simulink model "mrsMultiRobotAvoidance"  (R2018a)
settings: Solver=FixedStepAuto  StartTime=0.0  StopTime=inf  FixedStep=sampleTime  RelTol=1e-3
PreLoadFcn:
  | % Simulation parameters
  | load exampleMap
  | sampleTime = 0.05;
  | 
  | % Robot parameters
  | wheelRadius = 0.025;
  | robotRadius = 0.35;
  | 
  | % Lidar parameters
  | sensorOffset = [0,0];
  | scanAngles = linspace(-pi/2,pi/2,9)';
  | maxRange = 5;
libraries: mobileRoboticsLib x10
settings Model: EnablePacing=on  Creator=scastro  LastModifiedBy=scastro

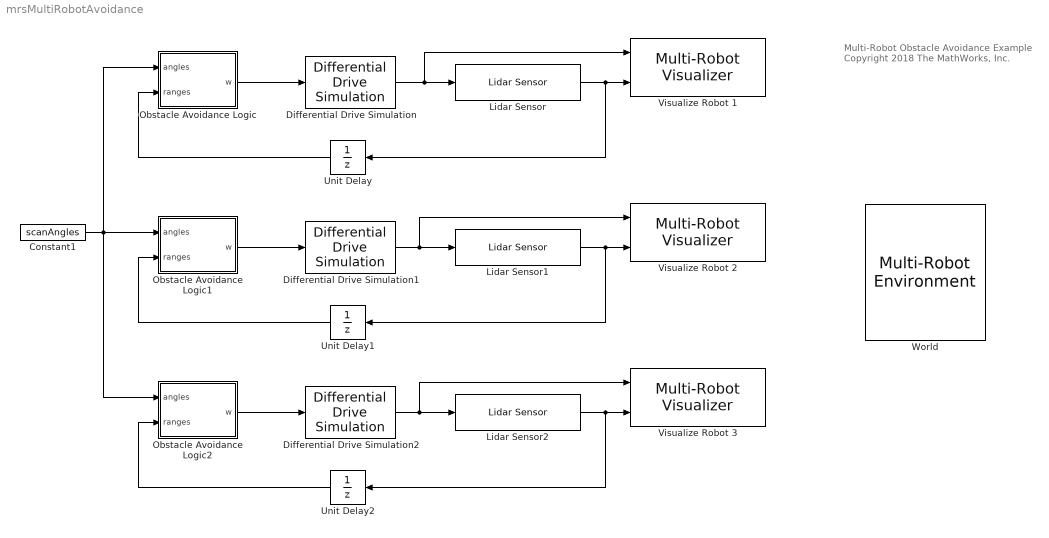
== system mrsMultiRobotAvoidance ==
  note: Multi-Robot Obstacle
      | Avoidance Example
      |
      | Copyright 2018 The MathWorks, Inc.
  Constant1 : Constant  Value=scanAngles
  Differential Drive Simulation : mobileRoboticsLib/Kinematic Models/Differential Drive/Differential Drive Simulation  OverrideUsingVariant=mode==2  wheelRadius=wheelRadius  wheelBase=robotRadius  initX=4  initY=4  initAngle=0  Ts=sampleTime
      settings: SourceProductName=Mobile Robotics Simulation Toolbox
  Differential Drive Simulation1 : mobileRoboticsLib/Kinematic Models/Differential Drive/Differential Drive Simulation  OverrideUsingVariant=mode==2  wheelRadius=wheelRadius  wheelBase=robotRadius  initX=8  initY=8  initAngle=pi/2  Ts=sampleTime
      settings: SourceProductName=Mobile Robotics Simulation Toolbox
  Differential Drive Simulation2 : mobileRoboticsLib/Kinematic Models/Differential Drive/Differential Drive Simulation  OverrideUsingVariant=mode==2  wheelRadius=wheelRadius  wheelBase=robotRadius  initX=7.5  initY=3  initAngle=-pi/4  Ts=sampleTime
      settings: SourceProductName=Mobile Robotics Simulation Toolbox
  Lidar Sensor : mobileRoboticsLib/Environments/Lidar Sensor  mapName=map  sensorOffset=sensorOffset  scanAngles=scanAngles  maxRange=maxRange  isMultiRobot=on  robotIdx=1
      settings: SourceProductName=Mobile Robotics Simulation Toolbox
  Lidar Sensor1 : mobileRoboticsLib/Environments/Lidar Sensor  mapName=map  sensorOffset=sensorOffset  scanAngles=scanAngles  maxRange=maxRange  isMultiRobot=on  robotIdx=2
      settings: SourceProductName=Mobile Robotics Simulation Toolbox
  Lidar Sensor2 : mobileRoboticsLib/Environments/Lidar Sensor  mapName=map  sensorOffset=sensorOffset  scanAngles=scanAngles  maxRange=maxRange  isMultiRobot=on  robotIdx=3
      settings: SourceProductName=Mobile Robotics Simulation Toolbox
  Obstacle Avoidance Logic : Stateflow chart  TreatAsAtomicUnit=on
  Obstacle Avoidance Logic1 : Stateflow chart  TreatAsAtomicUnit=on
  Obstacle Avoidance Logic2 : Stateflow chart  TreatAsAtomicUnit=on
  Unit Delay : UnitDelay  SampleTime=-1
  Unit Delay1 : UnitDelay  SampleTime=-1
  Unit Delay2 : UnitDelay  SampleTime=-1
  Visualize Robot 1 : mobileRoboticsLib/Environments/Multi-Robot Visualizer  idx=1  radius=robotRadius  showTraj=off  hasLidar=on  sensorOffset=sensorOffset  scanAngles=scanAngles  hasObjDetector=off  objDetectorOffset=[0;0]  objDetectorAngle=0  objDetectorFOV=pi/2  objDetectorMaxRange=5
      settings: SourceProductName=Mobile Robotics Simulation Toolbox
  Visualize Robot 2 : mobileRoboticsLib/Environments/Multi-Robot Visualizer  idx=2  radius=robotRadius  showTraj=off  hasLidar=on  sensorOffset=sensorOffset  scanAngles=scanAngles  hasObjDetector=off  objDetectorOffset=[0 0]  objDetectorAngle=0  objDetectorFOV=pi/2  objDetectorMaxRange=5
      settings: SourceProductName=Mobile Robotics Simulation Toolbox
  Visualize Robot 3 : mobileRoboticsLib/Environments/Multi-Robot Visualizer  idx=3  radius=robotRadius  showTraj=off  hasLidar=on  sensorOffset=sensorOffset  scanAngles=scanAngles  hasObjDetector=off  objDetectorOffset=[0 0]  objDetectorAngle=0  objDetectorFOV=pi/2  objDetectorMaxRange=5
      settings: SourceProductName=Mobile Robotics Simulation Toolbox
  World : mobileRoboticsLib/Environments/Multi-Robot Environment  numRobots=3  mapName=map  showWaypoints=off  showObjects=off  showRobotIds=on  plotSensorLines=on
      settings: SourceProductName=Mobile Robotics Simulation Toolbox
  wires:
  Differential Drive Simulation/1 -> Lidar Sensor/1, Visualize Robot 1/1
  Differential Drive Simulation1/1 -> Lidar Sensor1/1, Visualize Robot 2/1
  Obstacle Avoidance Logic/1(w) -> Differential Drive Simulation/1
  Unit Delay/1 -> Obstacle Avoidance Logic/2(ranges)
  Obstacle Avoidance Logic1/1(w) -> Differential Drive Simulation1/1
  Unit Delay1/1 -> Obstacle Avoidance Logic1/2(ranges)
  Unit Delay2/1 -> Obstacle Avoidance Logic2/2(ranges)
  Constant1/1 -> Obstacle Avoidance Logic2/1(angles), Obstacle Avoidance Logic1/1(angles), Obstacle Avoidance Logic/1(angles)
  Lidar Sensor2/1 -> Visualize Robot 3/2, Unit Delay2/1
  Obstacle Avoidance Logic2/1(w) -> Differential Drive Simulation2/1
  Differential Drive Simulation2/1 -> Lidar Sensor2/1, Visualize Robot 3/1
  Lidar Sensor/1 -> Unit Delay/1, Visualize Robot 1/2
  Lidar Sensor1/1 -> Unit Delay1/1, Visualize Robot 2/2

== stateflow chart mrsMultiRobotAvoidance/Obstacle Avoidance Logic1 ==
  state MainState [parallel]
    en,du:
    validIdx = ~isnan(ranges);
    validRanges = ranges(validIdx);
    validAngles = angles(validIdx);
    settings: executionOrder=1
    state Turn
      en,du:
      avgAngle = mean(validAngles./validRanges);
      state Left
        en, du:
        w = [0;12.5];
      state Right
        en, du:
        w = [12.5;0];
      (default) -> (junction 39)
      (junction 39) -> Left [order 1] : [avgAngle < 0]
      (junction 39) -> (junction 43) [order 2]
      Left -> Right : [after(1,sec) && ...
          | avgAngle > 0]
      Right -> Left : [after(1,sec) && ...
          | avgAngle < 0]
      (junction 43) -> Right
    state GoStraight
      en:
      w = [25; 25];
    (default) -> GoStraight
    GoStraight -> Turn : [any(validRanges<=1)]
    Turn -> GoStraight : [all(validRanges>1)]
  data: angles input; w output; ranges input; validRanges local size=numel(scanAngles); validIdx local; validAngles local size=numel(scanAngles); avgAngle local

== stateflow chart mrsMultiRobotAvoidance/Obstacle Avoidance Logic2 ==
  state MainState [parallel]
    en,du:
    validIdx = ~isnan(ranges);
    validRanges = ranges(validIdx);
    validAngles = angles(validIdx);
    settings: executionOrder=1
    state Turn
      en,du:
      avgAngle = mean(validAngles./validRanges);
      state Left
        en, du:
        w = [0;12.5];
      state Right
        en, du:
        w = [12.5;0];
      (default) -> (junction 39)
      (junction 39) -> Left [order 1] : [avgAngle < 0]
      (junction 39) -> (junction 43) [order 2]
      Left -> Right : [after(1,sec) && ...
          | avgAngle > 0]
      Right -> Left : [after(1,sec) && ...
          | avgAngle < 0]
      (junction 43) -> Right
    state GoStraight
      en:
      w = [25; 25];
    (default) -> GoStraight
    GoStraight -> Turn : [any(validRanges<=1)]
    Turn -> GoStraight : [all(validRanges>1)]
  data: angles input; w output; ranges input; validRanges local size=numel(scanAngles); validIdx local; validAngles local size=numel(scanAngles); avgAngle local

== stateflow chart mrsMultiRobotAvoidance/Obstacle Avoidance Logic ==
  state MainState [parallel]
    en,du:
    validIdx = ~isnan(ranges);
    validRanges = ranges(validIdx);
    validAngles = angles(validIdx);
    settings: executionOrder=1
    state Turn
      en,du:
      avgAngle = mean(validAngles./validRanges);
      state Left
        en, du:
        w = [0;12.5];
      state Right
        en, du:
        w = [12.5;0];
      (default) -> (junction 39)
      (junction 39) -> Left [order 1] : [avgAngle < 0]
      (junction 39) -> (junction 43) [order 2]
      Left -> Right : [after(1,sec) && ...
          | avgAngle > 0]
      Right -> Left : [after(1,sec) && ...
          | avgAngle < 0]
      (junction 43) -> Right
    state GoStraight
      en:
      w = [25; 25];
    (default) -> GoStraight
    GoStraight -> Turn : [any(validRanges<=1)]
    Turn -> GoStraight : [all(validRanges>1)]
  data: angles input; w output; ranges input; validRanges local size=numel(scanAngles); validIdx local; validAngles local size=numel(scanAngles); avgAngle local
